simulink model "Part3_NL"  (R2022a)
settings: Solver=VariableStepAuto  StartTime=0.0  StopTime=50  RelTol=1e-3
values from neighbouring files (symbols this model uses):
  D = diag([0.01, 0.01, 0.01])    [Driver_3.m]    (also in Driver_3NL.m)
  g = [0,0,-9.81]    [Driver_3.m]    (also in Driver_3NL.m)
  g2 = [0,0,0,-9.81]    [Driver_3.m]    (also in Driver_3NL.m)
  I = diag([3e-6, 3e-6, 1e-5])    [Driver_3.m]    (also in Driver_3NL.m)
  I_tf = diag([3e-6, 3e-6, 1e-5, 1])    [Driver_3.m]    (also in Driver_3NL.m)
  In = inv(I)    [Driver_3.m]    (also in Driver_3NL.m)
  k = 0.01    [Driver_3.m]    (also in Driver_3NL.m)
  K_d = 0.8    [Driver_3.m]    (also in Driver_3NL.m)
  K_i = 0.1    [Driver_3.m]    (also in Driver_3NL.m)
  K_p = 1.5    [Driver_3.m]    (also in Driver_3NL.m)
  m = 0.5    [Driver_3.m]    (also in Driver_3NL.m)
  mvec = [1 ... (first row only)    [Driver_3.m]    (also in Driver_3NL.m)
  TF2 = inv(tf2)    [Driver_3.m]    (also in Driver_3NL.m)
  tf_34 = [L*k, 0, -L*k, 0 ... (first row only)    [Driver_3.m]    (also in Driver_3NL.m)
undefined symbols (not defined in the file or in its folder): K_dxy, K_ixy, K_pxy, tf_xy, uxy, uzp
libraries: matrix_library x1
settings Model: Creator=askeo  LastModifiedBy=askeo

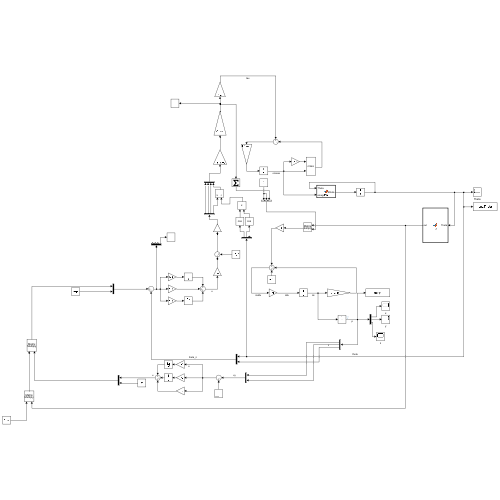
[thumbnail: Simulink's stored preview of the top-level diagram]
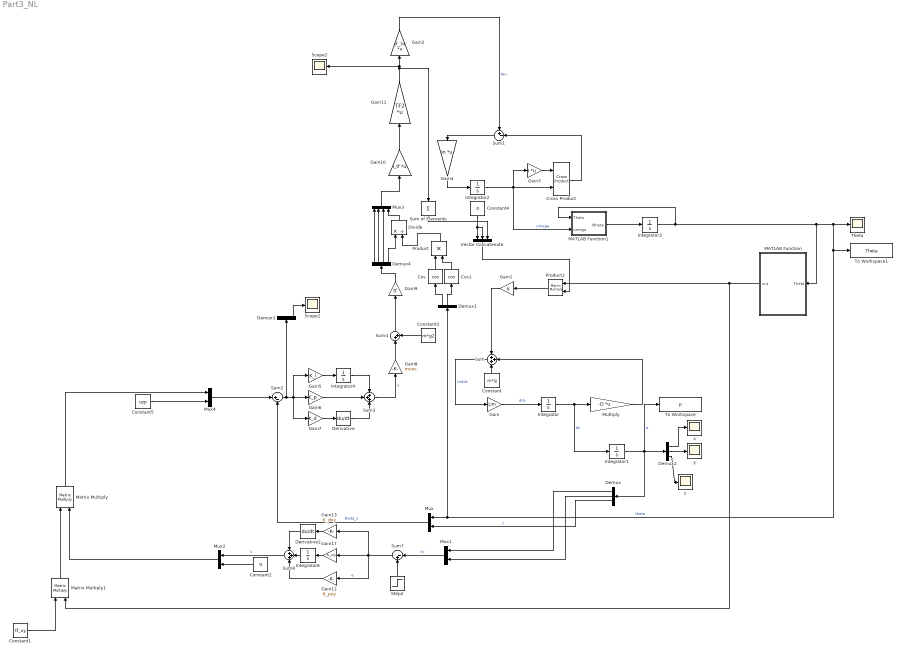
== system Part3_NL ==
  Constant : Constant  Value=m*g
  Constant1 : Constant  Value=tf_xy  VectorParams1D=off
  Constant2 : Constant  Value=0
  Constant3 : Constant  Value=m*g2
  Constant4 : Constant  Value=0
  Constant5 : Constant  Value=uzp
  Cos : Trigonometry  Operator=cos
  Cos1 : Trigonometry  Operator=cos
  Cross Product : matrix_library/Cross Product
      settings: SourceProductBaseCode=SL
  Demux : Demux  Outputs=3
  Demux1 : Demux  Outputs=3
  Demux2 : Demux  Outputs=3
  Demux3 : Demux
  Demux4 : Demux
  Derivative : Derivative
  Derivative2 : Derivative
  Divide : Product  Inputs=*/
  Gain : Gain  Gain=1/m
  Gain1 : Gain  Gain=k
  Gain10 : Gain  Gain=I_tf  Multiplication=Matrix(K*u) (u vector)
  Gain11 : Gain  Gain=TF2  Multiplication=Matrix(K*u) (u vector)
  Gain12 : Gain  Gain=K_pxy
  Gain13 : Gain  Gain=K_dxy
  Gain17 : Gain  Gain=K_ixy
  Gain2 : Gain  Gain=tf_34  Multiplication=Matrix(K*u) (u vector)
  Gain3 : Gain  Gain=I  Multiplication=Matrix(K*u) (u vector)
  Gain4 : Gain  Gain=In  Multiplication=Matrix(K*u) (u vector)
  Gain5 : Gain  Gain=K_i
  Gain6 : Gain  Gain=K_p
  Gain7 : Gain  Gain=K_d
  Gain8 : Gain  Gain=mvec
  Gain9 : Gain  Gain=tf
  Integrator : Integrator  InitialCondition=[0;0;0]
  Integrator1 : Integrator  InitialCondition=[0;0;0]
  Integrator2 : Integrator  InitialCondition=[0;0;0]
  Integrator3 : Integrator  InitialCondition=[0; 0; 0]
  Integrator4 : Integrator
  Integrator6 : Integrator
  MATLAB Function : MATLAB Function  TreatAsAtomicUnit=on
  MATLAB Function1 : MATLAB Function  TreatAsAtomicUnit=on
  Matrix Multiply : Product  Multiplication=Matrix(*)
  Matrix Multiply1 : Product  Multiplication=Matrix(*)
  Multiply : Gain  Gain=-D  Multiplication=Matrix(K*u) (u vector)
  Mux{,1..2,4} (4 alike) : Mux  Inputs=2
  Mux3 : Mux
  Product : Product
  Product2 : Product  Multiplication=Matrix(*)
  Scope1 : Scope
  Scope2 : Scope
  Step2 : Step  Time=0  After=uxy  SampleTime=0
  Sum : Sum  Inputs=+++
  Sum of Elements : Sum  Inputs=+
  Sum1 : Sum  Inputs=+-|
  Sum2 : Sum  Inputs=|+-
  Sum3 : Sum  Inputs=+++
  Sum4 : Sum  Inputs=|++
  Sum7 : Sum  Inputs=|-+
  Sum8 : Sum  Inputs=+++
  Theta : Scope
  To Workspace : ToWorkspace  VariableName=p  SampleTime=-1
  To Workspace1 : ToWorkspace  VariableName=Theta  SampleTime=0.001
  Vector Concatenate : Concatenate  NumInputs=3
  x : Scope
  y : Scope
  z : Scope
  wires:
  Integrator/1 -> Integrator1/1, Multiply/1  "dx"
  Gain2/1 -> Sum1/1  "tau"
  MATLAB Function1/1(dtheta) -> Integrator3/1
  Product/1 -> Divide/2
  Gain5/1 -> Integrator4/1
  Cos1/1 -> Product/2
  Gain8/1 -> Sum4/1
  Sum1/1 -> Gain4/1
  Integrator3/1 -> MATLAB Function/1(Theta), Mux/1, Demux1/1, To Workspace1/1, Theta/1, MATLAB Function1/1(Theta)  "theta"
  Cross Product/1 -> Sum1/2
  Demux3/4 -> Scope1/1
  Demux2/3 -> z/1
  Derivative/1 -> Sum3/3
  Gain11/1 -> Scope2/1, Gain2/1, Sum of Elements/1
  Integrator4/1 -> Sum3/1
  Constant/1 -> Sum/3
  Demux/3 -> Mux/2  "z"
  Gain6/1 -> Sum3/2
  Demux1/1 -> Cos/1
  Sum of Elements/1 -> Vector Concatenate/3
  Sum/1 -> Gain/1  "mddx"
  Gain1/1 -> Sum/1
  MATLAB Function/1(out) -> Matrix Multiply1/2, Product2/1
  Sum4/1 -> Gain9/1
  Gain10/1 -> Gain11/1
  Vector Concatenate/1 -> Product2/2
  Gain4/1 -> Integrator2/1
  Multiply/1 -> Sum/2
  Constant4/1 -> Vector Concatenate/2, Vector Concatenate/1
  Gain3/1 -> Cross Product/1
  Mux/1 -> Sum2/2  "theta_z"
  Constant3/1 -> Sum4/2
  Sum3/1 -> Gain8/1  "u"
  Gain/1 -> Integrator/1  "ddx"
  Product2/1 -> Gain1/1
  Demux1/2 -> Cos1/1
  Integrator1/1 -> Demux/1, Demux2/1, To Workspace/1  "p"
  Sum2/1 -> Gain6/1, Gain7/1, Gain5/1, Demux3/1
  Integrator2/1 -> MATLAB Function1/2(omega), Gain3/1, Cross Product/2  "omega"
  Gain7/1 -> Derivative/1
  Cos/1 -> Product/1
  Derivative2/1 -> Sum8/1
  Step2/1 -> Sum7/2
  Constant2/1 -> Mux2/2
  Sum8/1 -> Mux2/1  "u"
  Gain17/1 -> Integrator6/1
  Integrator6/1 -> Sum8/2
  Gain12/1 -> Sum8/3
  Demux/1 -> Mux1/1
  Mux2/1 -> Matrix Multiply/2
  Demux/2 -> Mux1/2
  Sum7/1 -> Gain13/1, Gain17/1, Gain12/1  "e"
  Mux1/1 -> Sum7/1  "xy"
  Constant5/1 -> Mux4/2
  Matrix Multiply/1 -> Mux4/1
  Matrix Multiply1/1 -> Matrix Multiply/1
  Constant1/1 -> Matrix Multiply1/1
  Gain13/1 -> Derivative2/1
  Demux2/2 -> y/1
  Demux2/1 -> x/1
  Gain9/1 -> Demux4/1
  Demux4/4 -> Divide/1
  Divide/1 -> Mux3/4
  Demux4/1 -> Mux3/1
  Demux4/2 -> Mux3/2
  Demux4/3 -> Mux3/3
  Mux3/1 -> Gain10/1
  Mux4/1 -> Sum2/1

== matlab function Part3_NL/MATLAB Function1 ==
  data: dtheta output; Theta input; omega input
function dtheta = fcn(Theta, omega)

C = [1, 0, -sin(Theta(2))
    0, cos(Theta(1)), cos(Theta(2))*sin(Theta(1))
    0, -sin(Theta(1)), cos(Theta(2))*cos(Theta(1))];

dtheta = inv(C)*omega;
end

== matlab function Part3_NL/MATLAB Function ==
  data: Theta input; out output
function out = Rb(Theta)

phi = Theta(1);
theta = Theta(2);
psi = Theta(3);

rbi = [cos(psi)*cos(theta), cos(psi)*sin(theta)*sin(phi) - sin(psi)*cos(phi), sin(psi)*sin(phi) + cos(psi)*sin(theta)*cos(phi)
    sin(psi)*cos(theta), cos(psi)*cos(phi) + sin(psi)*sin(theta)*sin(phi), sin(psi)*sin(theta)*sin(phi) - cos(psi)*sin(phi)
    -sin(theta), cos(theta)*sin(phi), cos(theta)*cos(phi)];

out = rbi;
end
